simulink model "MPC_planner_201105"  (R2020a)
settings: Solver=VariableStepAuto  StartTime=0  StopTime=30  FixedStep=0.001  RelTol=1e-3  AbsTol=1e-6
InitFcn:
  | Lw = 1.6;
  | lf = 1.4;
  | lr = 1.65;
values from neighbouring files (symbols this model uses):
  pos_error_max = 0.1    [nmpc_design.m]
  v_error_max = 0.12    [nmpc_design.m]
  yaw_error_max = 1.8*pi/180    (= 0.0314159265359)    [nmpc_design.m]
libraries: Solver_SF x1, mpclib x1
settings Model: ExtModeTrigMode=oneshot  ExtModeArmWhenConnect=off  OrderedModelArguments=off  Creator=ywata  LastModifiedBy=cksgh
settings SolverCC: AutoScaleAbsTol=off  AlgebraicLoopSolver=LineSearch
settings DataIOCC: SaveFormat=Array  ReturnWorkspaceOutputs=off  SignalLoggingName=sigsOut
settings OptimizationCC: BlockReduction=off  BooleanDataType=off  LifeSpan=inf
settings DebuggingCC: SaveWithParameterizedLinksMsg=none  UnderspecifiedInitializationDetection=Classic  MergeDetectMultiDrivingBlocksExec=none  SignalResolutionControl=TryResolveAllWithWarning  MultiTaskDSMMsg=warning  MultiTaskCondExecSysMsg=none  FcnCallInpInsideContextMsg=warning  StateNameClashWarn=warning  SFUnexpectedBacktrackingDiag=warning  SFNoUnconditionalDefaultTransitionDiag=warning  UnderSpecifiedDimensionMsg=warning  ArithmeticOperatorsInVariantConditions=warning
settings HardwareCC: ProdBitPerPointer=32  ProdBitPerSizeT=32  ProdBitPerPtrDiffT=32  ProdLargestAtomicFloat=None  ProdIntDivRoundTo=Undefined  ProdEndianess=Unspecified  ProdWordSize=32  ProdHWDeviceType=32-bit Generic  TargetUnknown=on
settings ModelReferenceCC: PropagateSignalLabelsOutOfModel=off
settings SFSimCC: SimUseLocalCustomCode=off  CustomCodeUndefinedFunction=UseInterfaceOnly
settings RTWCC: TemplateMakefile=grt_vc.tmf  RTWUseLocalCustomCode=off
settings CodeAppCC: StateflowObjectComments=on
settings GRTTargetCC: TargetFcnLib=ansi_tfl_tmw.mat  TargetLangStandard=C89/C90 (ANSI)  CombineOutputUpdateFcns=off  GRTInterface=on
settings ConfigComp: CovMetricSettings=dw  CovHtmlReporting=on  CovSaveCumulativeToWorkspaceVar=on  CovSaveSingleToWorkspaceVar=on  CovExternalEMLEnable=off

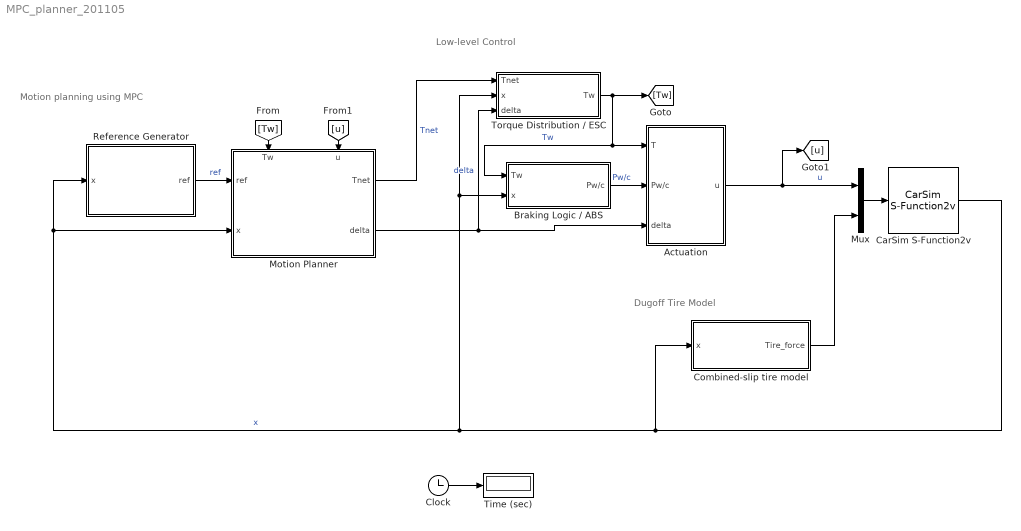
== system MPC_planner_201105 ==
  note: Dugoff Tire Model
  note: Low-level Control
  note: Motion planning using MPC
  Actuation : Subsystem
      mask Display: image('actuation_illust.png'); % Use "Edit Image" on toolstrip to change.
  Braking Logic / ABS : Subsystem
  CarSim S-Function2v : Solver_SF/CarSim S-Function2v  Priority=1  VehicleCode=i_i  SIMFILE=simfile.sim
      settings: AttributesFormatString=Vehicle Code: %<VehicleCode>
  Clock : Clock
  Combined-slip tire model : MATLAB Function  TreatAsAtomicUnit=on
  Motion Planner : Subsystem
      settings: PortSchema="{\"entries\":[{\"content\":{\"sides\":[{\"content\":{\"connectorIds\":[\"In1\",\"In2\"]},\"type\":\"ConnectorPlacement.EquallySpacedRectSide\",\"uuid\":\"a787b7cf-3cc5-479b-b22e-301a5134f3f2\"},{\"content\":{\"connectorIds\":[\"Out1\",\"Out2\"],\"side\":\"RIGHT\"},\"type\":\"ConnectorPlacement.EquallySpacedRectSide\",\"uuid\":\"a5bbac53-00df-45df-8e98-5eeb23656513\"},{\"content\":{\"connectorIds\":[\"In3\",\"In4\"],\"side\":\"TOP\"},\"type\":\"ConnectorPlacement.EquallySpacedRectSide\",\"uuid\":\"33a2ca21-4178-496c-88bb-777b57c1de4f\"}]},\"type\":\"ConnectorPlacement.EquallySpacedConnector\",\"uuid\":\"b7e07e24-f75d-4d53-b2e7-cf41caae1095\"}],\"packageUris\":[\"http://schema.mathworks.com/mf0/Connector/19700101\"],\"version\":\"1.0\"}"
      mask Display: image('mpc_illust.png'); % Use "Edit Image" on toolstrip to change.
  Mux : Mux  Inputs=[10 8]
  Reference Generator : Subsystem
      mask Display: image('refGen_illust.png'); % Use "Edit Image" on toolstrip to change.
  Time (sec) : Display
      settings: Format=bank  Decimation=100
  Torque Distribution / ESC : Subsystem
  wires:
  Clock/1 -> Time (sec)/1
  CarSim S-Function2v/1 -> Reference Generator/1(x), Motion Planner/2(x), Torque Distribution / ESC/2(x), Braking Logic / ABS/2(x), Combined-slip tire model/1(x)  "x"
  Reference Generator/1(ref) -> Motion Planner/1(ref)  "ref"
  Torque Distribution / ESC/1(Tw) -> [Tw], Actuation/1(T), Braking Logic / ABS/1(Tw)  "Tw"
  Braking Logic / ABS/1(Pw/c) -> Actuation/2(Pw/c)  "Pw/c"
  Mux/1 -> CarSim S-Function2v/1
  Actuation/1(u) -> [u], Mux/1  "u"
  Combined-slip tire model/1(Tire_force) -> Mux/2
  [u] -> Motion Planner/4(u)
  [Tw] -> Motion Planner/3(Tw)
  Motion Planner/2(delta) -> Torque Distribution / ESC/3(delta), Actuation/3(delta)  "delta"
  Motion Planner/1(Tnet) -> Torque Distribution / ESC/1(Tnet)  "Tnet"

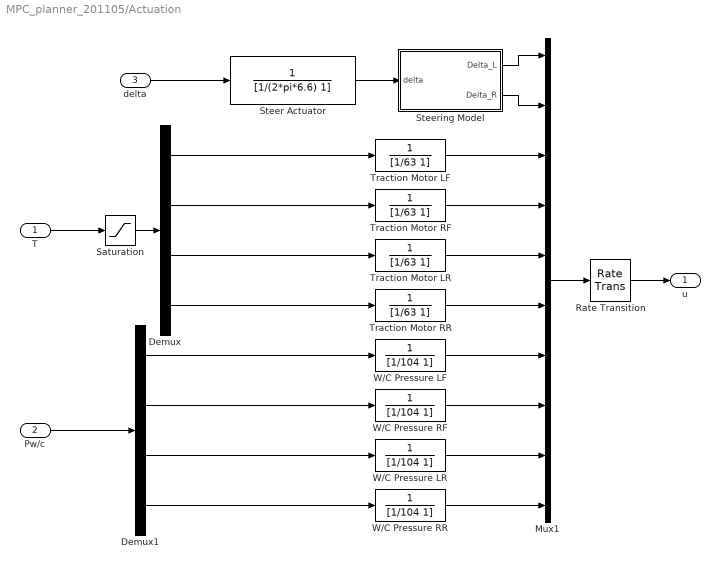
== system MPC_planner_201105/Actuation ==
  T : Inport
  Pw/c : Inport  Port=2
  delta : Inport  Port=3
  Demux : Demux
  Demux1 : Demux
  Mux1 : Mux  Inputs=10
  Rate Transition : RateTransition
  Saturation : Saturate  UpperLimit=650  LowerLimit=0
  Steer Actuator : TransferFcn  Denominator=[1/(2*pi*6.6) 1]
  Steering Model : Subsystem
  Traction Motor LF : TransferFcn  Denominator=[1/63 1]
  Traction Motor LR : TransferFcn  Denominator=[1/63 1]
  Traction Motor RF : TransferFcn  Denominator=[1/63 1]
  Traction Motor RR : TransferFcn  Denominator=[1/63 1]
  W/C Pressure LF : TransferFcn  Denominator=[1/104 1]
  W/C Pressure LR : TransferFcn  Denominator=[1/104 1]
  W/C Pressure RF : TransferFcn  Denominator=[1/104 1]
  W/C Pressure RR : TransferFcn  Denominator=[1/104 1]
  u : Outport
  wires:
  Rate Transition/1 -> u/1
  Traction Motor RR/1 -> Mux1/6
  Traction Motor LR/1 -> Mux1/5
  Traction Motor LF/1 -> Mux1/3
  Steering Model/2(Delta_R) -> Mux1/2
  Steering Model/1(Delta_L) -> Mux1/1
  Traction Motor RF/1 -> Mux1/4
  delta/1 -> Steer Actuator/1
  Mux1/1 -> Rate Transition/1
  Demux/1 -> Traction Motor LF/1
  Demux/2 -> Traction Motor RF/1
  Demux/3 -> Traction Motor LR/1
  Demux/4 -> Traction Motor RR/1
  Demux1/2 -> W/C Pressure RF/1
  W/C Pressure LF/1 -> Mux1/7
  W/C Pressure RF/1 -> Mux1/8
  W/C Pressure LR/1 -> Mux1/9
  W/C Pressure RR/1 -> Mux1/10
  Demux1/3 -> W/C Pressure LR/1
  Demux1/1 -> W/C Pressure LF/1
  Demux1/4 -> W/C Pressure RR/1
  Pw/c/1 -> Demux1/1
  Saturation/1 -> Demux/1
  T/1 -> Saturation/1
  Steer Actuator/1 -> Steering Model/1(delta)

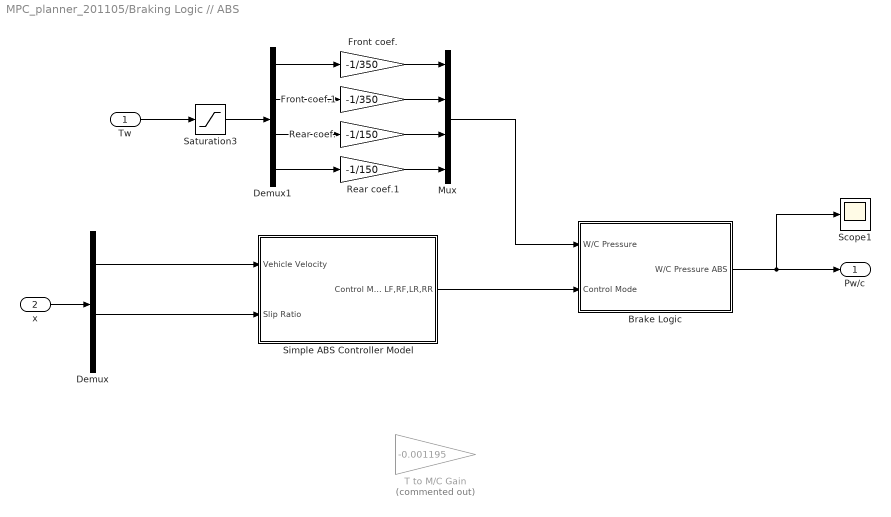
== system MPC_planner_201105/Braking Logic // ABS ==
  Tw : Inport
  x : Inport  Port=2
  "Brake Logic " : Subsystem
  Demux : Demux  Outputs=[5 1 3 4 1 4]
  Demux1 : Demux
  Front coef. : Gain  Gain=-1/350
  Front coef.1 : Gain  Gain=-1/350
  Mux : Mux
  Rear coef. : Gain  Gain=-1/150
  Rear coef.1 : Gain  Gain=-1/150
  Saturation3 : Saturate  UpperLimit=0  LowerLimit=-2300/4
  Scope1 : Scope
  Simple ABS Controller Model : Subsystem
  T to M/C Gain : Gain  Commented=on  Gain=-0.001195
  Pw/c : Outport
  wires:
  x/1 -> Demux/1
  Mux/1 -> "Brake Logic "/1(W/C Pressure)
  Demux/2 -> Simple ABS Controller Model/1(Vehicle Velocity)
  Demux/4 -> Simple ABS Controller Model/2(Slip Ratio)
  Simple ABS Controller Model/1(Control Mode LF,RF,LR,RR) -> "Brake Logic "/2(Control Mode)
  Tw/1 -> Saturation3/1
  Front coef.1/1 -> Mux/2
  Front coef./1 -> Mux/1
  Rear coef./1 -> Mux/3
  Rear coef.1/1 -> Mux/4
  Demux1/1 -> Front coef./1
  Demux1/2 -> Front coef.1/1
  Demux1/3 -> Rear coef./1
  Demux1/4 -> Rear coef.1/1
  "Brake Logic "/1(W/C Pressure ABS) -> Scope1/1, Pw/c/1
  Saturation3/1 -> Demux1/1

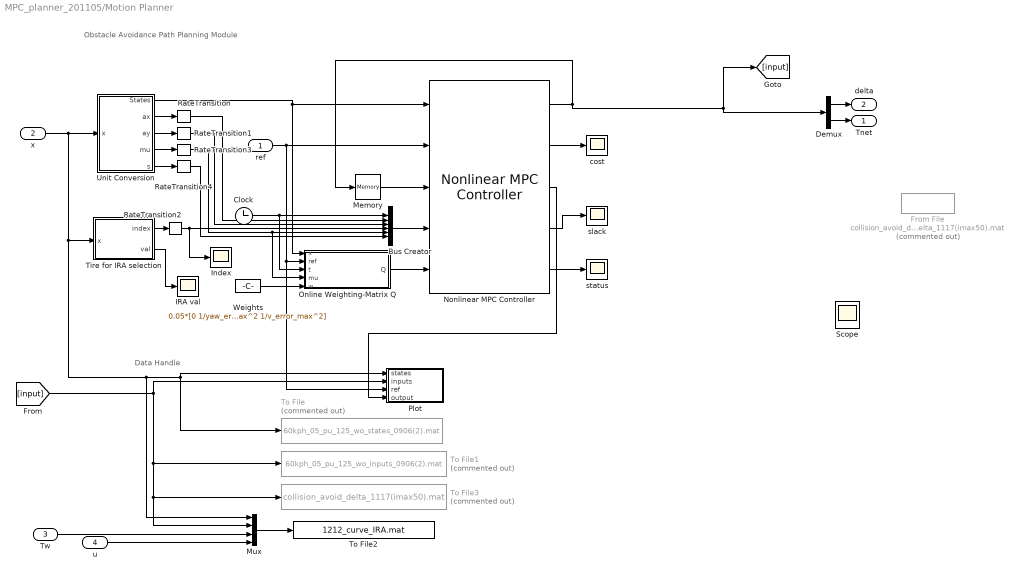
== system MPC_planner_201105/Motion Planner ==
  note: Data Handle
  note: Obstacle Avoidance Path Planning Module
  ref : Inport
  x : Inport  Port=2
  Tw : Inport  Port=3
  u : Inport  Port=4
  Bus Creator : BusCreator  Inputs=6  OutDataTypeStr=Bus: myBusObject  NonVirtualBus=on
      settings: InheritFromInputs=off
  Clock : Clock
  Demux : Demux  Outputs=2
  From File : FromFile  Commented=on  FileName=collision_avoid_delta_1117(imax50).mat  SampleTime=0
  IRA val : Scope
  Index : Scope
  Memory : Memory  InitialCondition=[0 100]  InheritSampleTime=on
  Mux : Mux
  Nonlinear MPC Controller : mpclib/Nonlinear MPC Controller  SCDEnableBlockLinearizationSpecification=on  nlmpcobj=nlobj  UseObjectTs=on  UseMEX=off  md_enabled=off  mvtarget_enabled=off  param_enabled=on  cost_enabled=on  mvseq_enabled=off  stateseq_enabled=off  ovseq_enabled=on  slack_enabled=on  status_enabled=on  ov_min=off  ov_max=off  mv_min=off  mv_max=off  mvrate_min=off  mvrate_max=off  state_min=off  state_max=off  ov_weight=on  mv_weight=off  mvrate_weight=off  ecr_weight=off  nlp_initialize=off
  Online Weighting-Matrix Q : MATLAB Function  TreatAsAtomicUnit=on  SystemSampleTime=0.05
  Plot : Subsystem
  RateTransition : RateTransition
  RateTransition1 : RateTransition
  RateTransition2 : RateTransition  InitialCondition=1
  RateTransition3 : RateTransition  InitialCondition=0.9
  RateTransition4 : RateTransition  InitialCondition=[0 0 0 0]'
  Scope : Scope
  Tire for IRA selection : MATLAB Function  TreatAsAtomicUnit=on
  To File : ToFile  Commented=on  Filename=60kph_05_pu_125_wo_states_0906(2).mat  MatrixName=states  SaveFormat=Timeseries
  To File1 : ToFile  Commented=on  Filename=60kph_05_pu_125_wo_inputs_0906(2).mat  MatrixName=inputs  SaveFormat=Timeseries
  To File2 : ToFile  Filename=1212_curve_IRA.mat  MatrixName=data  SaveFormat=Timeseries
  To File3 : ToFile  Commented=on  Filename=collision_avoid_delta_1117(imax50).mat  MatrixName=inputs  SaveFormat=Timeseries
  Unit Conversion : Subsystem
  Weights : Constant  Value=0.05*[0 1/yaw_error_max^2 1/pos_error_max^2 1/pos_error_max^2 1/v_error_max^2]
  cost : Scope
  slack : Scope
  status : Scope
  Tnet : Outport
  delta : Outport  Port=2
  wires:
  Memory/1 -> Nonlinear MPC Controller/3
  ref/1 -> Plot/3(ref), Online Weighting-Matrix Q/2(ref), Nonlinear MPC Controller/2
  Unit Conversion/1(States) -> Online Weighting-Matrix Q/1(x), Nonlinear MPC Controller/1
  Nonlinear MPC Controller/5 -> status/1
  Nonlinear MPC Controller/2 -> cost/1
  Clock/1 -> Online Weighting-Matrix Q/3(t), Bus Creator/1
  RateTransition/1 -> Bus Creator/2
  RateTransition1/1 -> Bus Creator/3
  Unit Conversion/4(mu) -> RateTransition3/1
  Bus Creator/1 -> Nonlinear MPC Controller/4
  Unit Conversion/2(ax) -> RateTransition/1
  Weights/1 -> Online Weighting-Matrix Q/5(w)
  x/1 -> Mux/1, To File/1, Plot/1(states), Tire for IRA selection/1(x), Unit Conversion/1(x)
  Unit Conversion/3(ay) -> RateTransition1/1
  RateTransition2/1 -> Index/1, Bus Creator/4
  Nonlinear MPC Controller/4 -> slack/1
  Demux/2 -> Tnet/1
  Demux/1 -> delta/1
  Nonlinear MPC Controller/1 -> Demux/1, [input], Memory/1
  [input] -> Mux/2, To File3/1, To File1/1, Plot/2(inputs)
  RateTransition3/1 -> Online Weighting-Matrix Q/4(mu), Bus Creator/5
  Unit Conversion/5(s) -> RateTransition4/1
  RateTransition4/1 -> Bus Creator/6
  Mux/1 -> To File2/1
  Tire for IRA selection/1(index) -> RateTransition2/1
  Tw/1 -> Mux/3
  u/1 -> Mux/4
  Online Weighting-Matrix Q/1(Q) -> Nonlinear MPC Controller/5
  Nonlinear MPC Controller/3 -> Plot/4(output)
  Tire for IRA selection/2(val) -> IRA val/1

== system MPC_planner_201105/Reference Generator ==
  x : Inport
  MATLAB Function : MATLAB Function  TreatAsAtomicUnit=on  SystemSampleTime=0.05
  Spline curve from workspace : FromWorkspace  Commented=on  VariableName=s
  ref : Outport
  wires:
  MATLAB Function/1(ref) -> ref/1
  x/1 -> MATLAB Function/1(state)

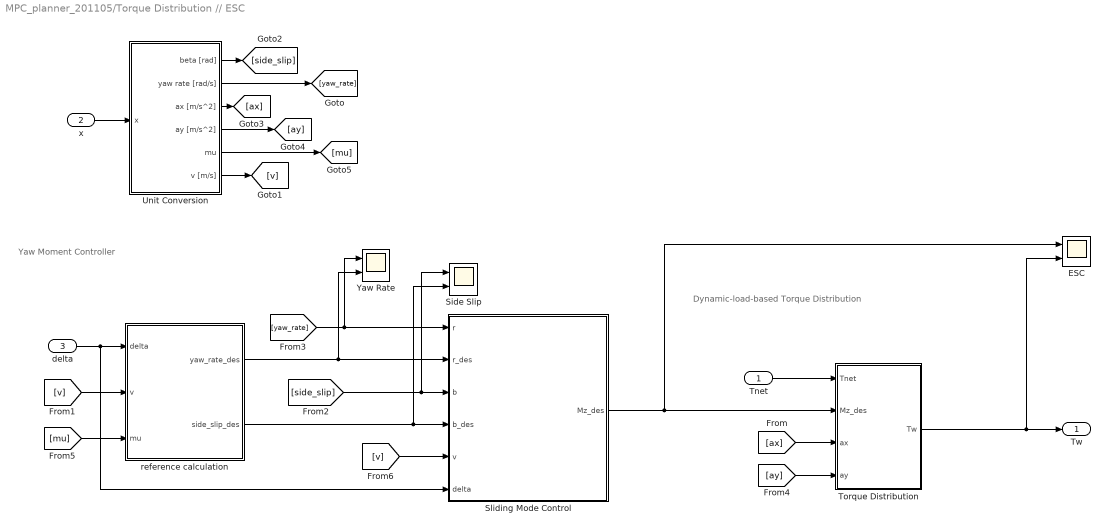
== system MPC_planner_201105/Torque Distribution // ESC ==
  note: Dynamic-load-based Torque Distribution
  note: Yaw Moment Controller
  Tnet : Inport
  x : Inport  Port=2
  delta : Inport  Port=3
  ESC : Scope  NumInputPorts=2
  Side Slip : Scope  NumInputPorts=2
  Sliding Mode Control : MATLAB Function  TreatAsAtomicUnit=on
  Torque Distribution : MATLAB Function  TreatAsAtomicUnit=on
  Unit Conversion : Subsystem
  Yaw Rate : Scope  NumInputPorts=2
  reference calculation : MATLAB Function  TreatAsAtomicUnit=on
  Tw : Outport
  wires:
  [yaw_rate] -> Yaw Rate/1, Sliding Mode Control/1(r)
  delta/1 -> reference calculation/1(delta), Sliding Mode Control/6(delta)
  reference calculation/2(side_slip_des) -> Side Slip/2, Sliding Mode Control/4(b_des)
  reference calculation/1(yaw_rate_des) -> Yaw Rate/2, Sliding Mode Control/2(r_des)
  [side_slip] -> Side Slip/1, Sliding Mode Control/3(b)
  [v] -> reference calculation/2(v)
  x/1 -> Unit Conversion/1(x)
  Unit Conversion/2(yaw rate [rad/s]) -> [yaw_rate]
  Unit Conversion/1(beta [rad]) -> [side_slip]
  Unit Conversion/3(ax [m/s^2]) -> [ax]
  Unit Conversion/4(ay [m/s^2]) -> [ay]
  [ay] -> Torque Distribution/4(ay)
  [ax] -> Torque Distribution/3(ax)
  Torque Distribution/1(Tw) -> ESC/2, Tw/1
  Tnet/1 -> Torque Distribution/1(Tnet)
  Unit Conversion/5(mu) -> [mu]
  [mu] -> reference calculation/3(mu)
  Unit Conversion/6(v [m/s]) -> [v]
  [v] -> Sliding Mode Control/5(v)
  Sliding Mode Control/1(Mz_des) -> Torque Distribution/2(Mz_des), ESC/1

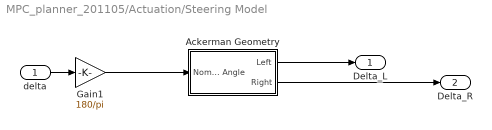
== system MPC_planner_201105/Actuation/Steering Model ==
  delta : Inport
  Ackerman Geometry : Subsystem
  Gain1 : Gain  Gain=180/pi
  Delta_L : Outport
  Delta_R : Outport  Port=2
  wires:
  Ackerman Geometry/2(Right) -> Delta_R/1
  Gain1/1 -> Ackerman Geometry/1(Nominal Angle)
  Ackerman Geometry/1(Left) -> Delta_L/1
  delta/1 -> Gain1/1

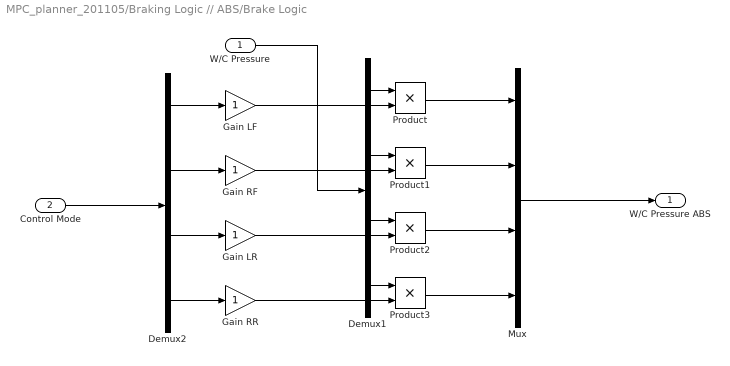
== system MPC_planner_201105/Braking Logic // ABS/Brake Logic  ==
  W/C Pressure : Inport
  Control Mode : Inport  Port=2
  Demux1 : Demux
  Demux2 : Demux
  Gain LF : Gain
  Gain LR : Gain
  Gain RF : Gain
  Gain RR : Gain
  Mux : Mux
  Product{,1..3} (4 alike) : Product
  W/C Pressure ABS : Outport
  wires:
  Demux2/1 -> Gain LF/1
  Demux2/4 -> Gain RR/1
  Demux2/3 -> Gain LR/1
  Gain LR/1 -> Product2/2
  Mux/1 -> W/C Pressure ABS/1
  Gain RF/1 -> Product1/2
  Gain RR/1 -> Product3/2
  Demux2/2 -> Gain RF/1
  Gain LF/1 -> Product/2
  Control Mode/1 -> Demux2/1
  Product/1 -> Mux/1
  Product1/1 -> Mux/2
  Product2/1 -> Mux/3
  Product3/1 -> Mux/4
  Demux1/1 -> Product/1
  Demux1/2 -> Product1/1
  Demux1/3 -> Product2/1
  Demux1/4 -> Product3/1
  W/C Pressure/1 -> Demux1/1

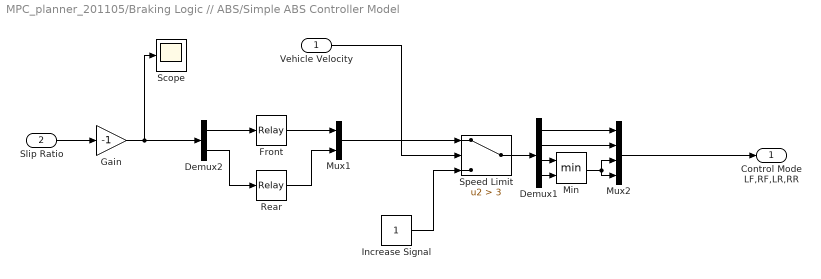
== system MPC_planner_201105/Braking Logic // ABS/Simple ABS Controller Model ==
  Vehicle Velocity : Inport
  Slip Ratio : Inport  Port=2
  Demux1 : Demux
  Demux2 : Demux  Outputs=[2 2]
  Front : Relay  OnSwitchValue=0.1  OffSwitchValue=0.05  OnOutputValue=0  OffOutputValue=1
  Gain : Gain  Gain=-1
  Increase Signal : Constant
  Min : MinMax  Inputs=2
  Mux1 : Mux  Inputs=2
  Mux2 : Mux
  Rear : Relay  OnSwitchValue=0.1  OffSwitchValue=0.05  OnOutputValue=0  OffOutputValue=1
  Scope : Scope
  Speed Limit : Switch  Criteria=u2 > Threshold  Threshold=3
  Control Mode LF,RF,LR,RR : Outport
  wires:
  Front/1 -> Mux1/1
  Speed Limit/1 -> Demux1/1
  Min/1 -> Mux2/3, Mux2/4
  Mux1/1 -> Speed Limit/1
  Increase Signal/1 -> Speed Limit/3
  Demux1/2 -> Mux2/2
  Demux1/4 -> Min/2
  Vehicle Velocity/1 -> Speed Limit/2
  Rear/1 -> Mux1/2
  Demux1/3 -> Min/1
  Demux1/1 -> Mux2/1
  Mux2/1 -> Control Mode LF,RF,LR,RR/1
  Slip Ratio/1 -> Gain/1
  Demux2/1 -> Front/1
  Demux2/2 -> Rear/1
  Gain/1 -> Scope/1, Demux2/1

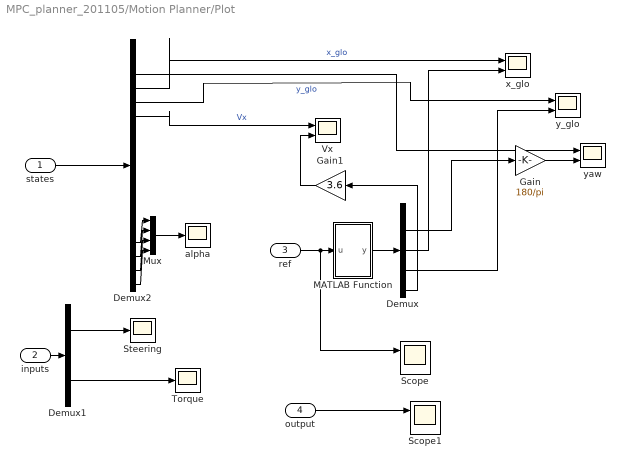
== system MPC_planner_201105/Motion Planner/Plot ==
  states : Inport
  inputs : Inport  Port=2
  ref : Inport  Port=3
  output : Inport  Port=4
  Demux : Demux  Outputs=5
  Demux1 : Demux  Outputs=2
  Demux2 : Demux  Outputs=18
  Gain : Gain  Gain=180/pi
  Gain1 : Gain  Gain=3.6
  MATLAB Function : MATLAB Function  TreatAsAtomicUnit=on
  Mux : Mux
  Scope : Scope  NumInputPorts=2
  Scope1 : Scope  NumInputPorts=2
  Steering : Scope
  Torque : Scope
  Vx : Scope  NumInputPorts=2
  alpha : Scope
  x_glo : Scope  NumInputPorts=2
  y_glo : Scope  NumInputPorts=2
  yaw : Scope  NumInputPorts=2
  wires:
  states/1 -> Demux2/1
  Demux2/5 -> y_glo/1  "y_glo"
  Demux2/6 -> Vx/1  "Vx"
  inputs/1 -> Demux1/1
  Demux1/1 -> Steering/1
  Demux1/2 -> Torque/1
  Demux2/15 -> Mux/1
  Demux2/16 -> Mux/2
  Demux2/17 -> Mux/3
  Demux2/18 -> Mux/4
  Mux/1 -> alpha/1
  Demux/4 -> y_glo/2
  MATLAB Function/1(y) -> Demux/1
  ref/1 -> Scope/1, MATLAB Function/1(u)
  Demux2/3 -> yaw/1
  Demux/2 -> Gain/1
  Demux2/4 -> x_glo/1  "x_glo"
  Demux/3 -> x_glo/2
  Gain/1 -> yaw/2
  Demux/5 -> Gain1/1
  Gain1/1 -> Vx/2
  output/1 -> Scope1/1

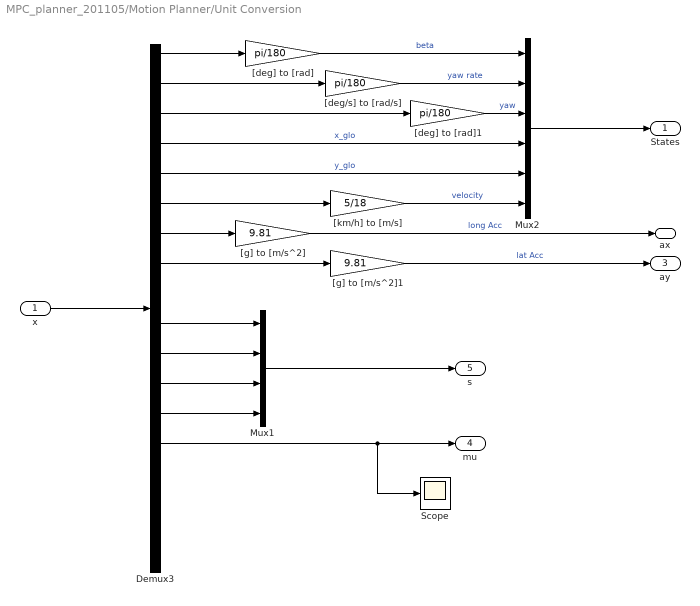
== system MPC_planner_201105/Motion Planner/Unit Conversion ==
  x : Inport
  Demux3 : Demux  Outputs=18
  Mux1 : Mux
  Mux2 : Mux  Inputs=6
  Scope : Scope
  "[deg/s] to [rad/s]" : Gain  Gain=pi/180
  "[deg] to [rad]" : Gain  Gain=pi/180
  "[deg] to [rad]1" : Gain  Gain=pi/180
  "[g] to [m/s^2]" : Gain  Gain=9.81
  "[g] to [m/s^2]1" : Gain  Gain=9.81
  "[km/h] to [m/s]" : Gain  Gain=5/18
  States : Outport
  ax : Outport  Port=2
  ay : Outport  Port=3
  mu : Outport  Port=4
  s : Outport  Port=5
  wires:
  Demux3/1 -> "[deg] to [rad]"/1
  x/1 -> Demux3/1
  "[km/h] to [m/s]"/1 -> Mux2/6  "velocity"
  Mux2/1 -> States/1
  Demux3/6 -> "[km/h] to [m/s]"/1
  "[deg] to [rad]"/1 -> Mux2/1  "beta"
  Demux3/2 -> "[deg/s] to [rad/s]"/1
  "[deg/s] to [rad/s]"/1 -> Mux2/2  "yaw rate"
  Demux3/3 -> "[deg] to [rad]1"/1
  "[deg] to [rad]1"/1 -> Mux2/3  "yaw"
  Demux3/4 -> Mux2/4  "x_glo"
  Demux3/5 -> Mux2/5  "y_glo"
  Demux3/7 -> "[g] to [m/s^2]"/1
  "[g] to [m/s^2]"/1 -> ax/1  "long Acc"
  Demux3/8 -> "[g] to [m/s^2]1"/1
  "[g] to [m/s^2]1"/1 -> ay/1  "lat Acc"
  Demux3/14 -> Scope/1, mu/1
  Demux3/10 -> Mux1/1
  Demux3/11 -> Mux1/2
  Demux3/12 -> Mux1/3
  Demux3/13 -> Mux1/4
  Mux1/1 -> s/1

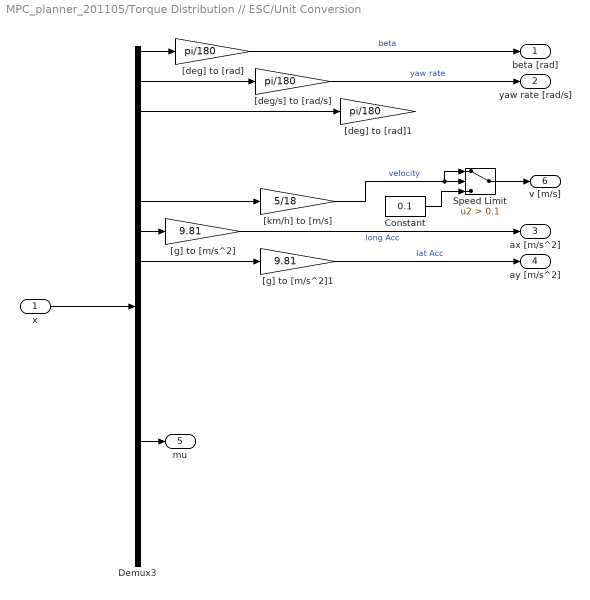
== system MPC_planner_201105/Torque Distribution // ESC/Unit Conversion ==
  x : Inport
  Constant : Constant  Value=0.1
  Demux3 : Demux  Outputs=18
  Speed Limit : Switch  Criteria=u2 > Threshold  Threshold=0.1
  "[deg/s] to [rad/s]" : Gain  Gain=pi/180
  "[deg] to [rad]" : Gain  Gain=pi/180
  "[deg] to [rad]1" : Gain  Gain=pi/180
  "[g] to [m/s^2]" : Gain  Gain=9.81
  "[g] to [m/s^2]1" : Gain  Gain=9.81
  "[km/h] to [m/s]" : Gain  Gain=5/18
  beta [rad] : Outport
  yaw rate [rad/s] : Outport  Port=2
  ax [m/s^2] : Outport  Port=3
  ay [m/s^2] : Outport  Port=4
  mu : Outport  Port=5
  v [m/s] : Outport  Port=6
  wires:
  Demux3/1 -> "[deg] to [rad]"/1
  x/1 -> Demux3/1
  "[km/h] to [m/s]"/1 -> Speed Limit/1, Speed Limit/2  "velocity"
  Demux3/6 -> "[km/h] to [m/s]"/1
  "[deg] to [rad]"/1 -> beta [rad]/1  "beta"
  Demux3/2 -> "[deg/s] to [rad/s]"/1
  "[deg/s] to [rad/s]"/1 -> yaw rate [rad/s]/1  "yaw rate"
  Demux3/3 -> "[deg] to [rad]1"/1
  Demux3/7 -> "[g] to [m/s^2]"/1
  "[g] to [m/s^2]"/1 -> ax [m/s^2]/1  "long Acc"
  Demux3/8 -> "[g] to [m/s^2]1"/1
  "[g] to [m/s^2]1"/1 -> ay [m/s^2]/1  "lat Acc"
  Demux3/14 -> mu/1
  Constant/1 -> Speed Limit/3
  Speed Limit/1 -> v [m/s]/1

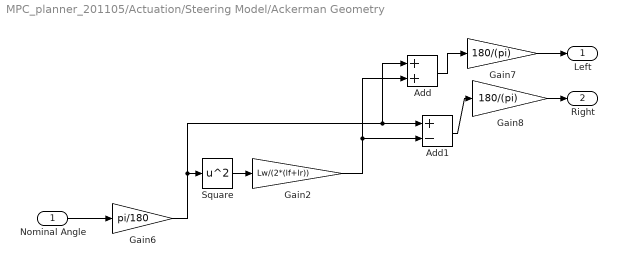
== system MPC_planner_201105/Actuation/Steering Model/Ackerman Geometry ==
  Nominal Angle : Inport
  Add : Sum
  Add1 : Sum  Inputs=+-
  Gain2 : Gain  Gain=Lw/(2*(lf+lr))
  Gain6 : Gain  Gain=pi/180
  Gain7 : Gain  Gain=180/(pi)
  Gain8 : Gain  Gain=180/(pi)
  Square : Math  Operator=square  SignedPower=on  SaturateOnIntegerOverflow=on
  Left : Outport
  Right : Outport  Port=2
  wires:
  Square/1 -> Gain2/1
  Gain6/1 -> Add/1, Add1/1, Square/1
  Add/1 -> Gain7/1
  Add1/1 -> Gain8/1
  Nominal Angle/1 -> Gain6/1
  Gain7/1 -> Left/1
  Gain8/1 -> Right/1
  Gain2/1 -> Add1/2, Add/2

== matlab function MPC_planner_201105/Torque Distribution // ESC/Sliding Mode Control ==
  data: r input; Mz_des output; r_des input; b input; b_des input; v input; delta input
function Mz_des  = fcn(r,r_des,b,b_des, v, delta)

m = 1650 + 180; % Sprung mass and unsprung mass
Iz = 3234;
lf = 1.4;
lr = 1.65;

% norminal cornering stiffness [N/rad]
Cf = -(1305.3)*180/pi/7; % Fzf = 4856*2 N
Cr = -(1122.7)*180/pi/7; % Fzr = 4140*2 N


% Yaw moment input based on sliding mode control
rho = 0.001;
K = 3;
theta = 100;
a11 = -2*(Cf+Cr)/(m*v);
a12 = -1-2*(lf*Cf-lr*Cr)/(m*v^2);
a21 = -2*(lf*Cf-lr*Cr)/Iz;
a22 = -2*(lf^2*Cf+lr^2*Cr)/(Iz*v);

Mz_eq = -Iz*(rho*a11+a21)*b-Iz*(rho*a12+a22)*r-Iz*(rho*2*Cf/m/v+2*lf*Cf/Iz)*delta;
% Mz_eq = -Iz*(a21*b+a22*r+2*lf*Cf/Iz)*delta;
e = ((r-r_des) +rho*(b-b_des) ) / theta;
if abs(e) > 1
    e = sign(e);
end

Mz_des = Mz_eq - Iz*(K*e);
% Mz_des = Mz_des*0.001;

== matlab function MPC_planner_201105/Torque Distribution // ESC/reference calculation ==
  data: delta input; yaw_rate_des output; v input; side_slip_des output; mu input
function [yaw_rate_des, side_slip_des] = fcn(delta, v, mu)

m = 1650 + 180; % Sprung mass and unsprung mass
g = 9.81;
lf = 1.4;
lr = 1.65;
L = lf+lr;

% cornering stiffness [N/rad]
Cf = -1305.3 * 180/pi/7; % Fzf = 4856*2 N
Cr = -1122.7 * 180/pi/7; % Fzr = 4140*2 N

% desired Yaw rate and Side slip
yaw_rate_des = sign(delta)*abs(v/(lf+lr+ (m*v^2*(lr*Cr-lf*Cf)/(2*Cf*Cr*L)) )*delta); % [rad/s]
side_slip_des = sign(delta)*abs((lr-lf*m*v^2/(2*Cr*L))/(L+(m*v^2*(lr*Cr-lf*Cf)/(2*Cf*Cr*L)))*delta); % [rad]

% upper bounnd
yaw_rate_ub = abs(0.85*mu*g/v);
side_slip_ub = abs(atan(0.02*mu*9.81));

if abs(yaw_rate_des) > yaw_rate_ub
    yaw_rate_des = sign(delta)*yaw_rate_ub;
end
if abs(side_slip_des) > side_slip_ub
    side_slip_des = sign(delta)*side_slip_ub;
end
side_slip_des = -side_slip_des;

== matlab function MPC_planner_201105/Motion Planner/Online Weighting-Matrix Q ==
  data: x input; ref input; t input; mu input; Q output; w input
function Q = fcn(x,ref,t,mu,w)
x_ref = ref(:,3);
y_ref = ref(:,4);
V = x(6);
g = 9.81;
p = 20;
Ts = 0.05;

af = 6*sqrt(2)/2; b = 3*sqrt(2)/2;
d = V.^2/mu/g - 2;
v_obs = 50/3.6;
x_ini = 70;
x_obs_cur = x_ini + t*v_obs;

%%%% Moving obstacle %%%%
% x_obs = (x_obs_cur+v_obs*Ts: v_obs*Ts :x_obs_cur + v_obs*Ts*p)';
% if x_ref(1) < x_obs_cur
%     K_mv = ( (x_ref - x_obs).^2./d.^2 + (y_ref+2).^2./b^2 ).^0.5 - 1;
%     J_mv = (exp(-0.1*K_mv)./max(K_mv,1e-2));
% else
%     K_mv = ( (x_ref - x_obs).^2./af.^2 + (y_ref+2).^2./b^2 ).^0.5 - 1;
%     J_mv = (exp(-0.1*K_mv)./max(K_mv,1e-2));
% end
%%%%%%%%%%%%%%%%%%%%%%%%%%
p_obs = [70 -2];

%%%% Pop-up obstacle %%%%
J_mv = zeros(p,1);
% if x_ref(1) > 70-2-44.444
%     if x_ref(1) < x_obs_cur
%         d = 70 - x_ref(1) -2 ;
%         K_mv = ( (x_ref - p_obs(1)).^2./d.^2 + (y_ref - p_obs(2)).^2./b^2 ).^0.5 - 1;
%         J_mv = 0.1*(exp(-10*K_mv)./max(K_mv,1e-7));
%     else
%         K_mv = ( (x_ref - p_obs(1)).^2./af.^2 + (y_ref - p_obs(2)).^2./b^2 ).^0.5 - 1;
%         J_mv = 0.1*(exp(-10*K_mv)./max(K_mv,1e-7));
%     end
% end
%%%%%%%%%%%%%%%%%%%%%%%%



%%%%%%%%%%%%%%%%%%%%% Popup Obstacle curve %%%%%%%%%%%%%%%%%%%%%%
if y_ref(1) >= 32 %29.17
    if y_ref(1) < 52
        d = p_obs(2) - y_ref(1)-2;
        K_obs = ( (x_ref - p_obs(1)).^2./b^2 + (y_ref-p_obs(2)).^2./d^2 ).^0.5 - 1;
        J_mv = 0.1*(exp(-10*K_obs)./max(K_obs,1e-7));
    else
        K_obs = ( (x_ref - p_obs(1)).^2./b^2 + (y_ref-p_obs(2)).^2./af^2 ).^0.5 - 1;
        J_mv = 0.1*(exp(-10*K_obs)./max(K_obs,1e-7));
    end
end
%%%%%%%%%%%%%%%%%%%%%%%%%%%%%%%%%%%%%%%%%%%%%%%%%%%%%%%%%%%%
k = 1./(1+0.1*J_mv);
Q = [zeros(p,1) w(2)*ones(p,1).*k w(3)*ones(p,1).*k w(4)*ones(p,1).*k w(5)*ones(p,1)];

== matlab function MPC_planner_201105/Reference Generator/MATLAB Function ==
  data: ref output; state input
function ref = fcn(state)
Hp = 20; Ts = 0.05;
ref = zeros(Hp,5);

%%%%%%%%%%%%%%%%%%%%%%%%%%% CURVE Scenario %%%%%%%%%%%%%%%%%%%%%%%%%%%%%%%%

% Load reference data
y = load('curve_left_R50_y-s.mat');
x = load('curve_left_R50_x-s.mat');
v = load('v_profile_cur50_0.3_v-s.mat');
y = y.y;
x = x.x;
v = v.v;

% initialize
x_glo = state(4); y_glo = state(5);
s = sqrt(x_glo^2 + y_glo^2); ds = 0.01;
x_ref_init = x(int16(s/ds));
y_ref_init = y(int16(s/ds));
Hp = 20; Ts = 0.05;


% Search shortest point of reference
d = dis(x_glo,y_glo,x_ref_init,y_ref_init);
df = dis(x_glo,y_glo,x(int16(s/ds) + 2),y(int16(s/ds) + 2)); % Forward search
db = dis(x_glo,y_glo,x(int16(s/ds) - 2),y(int16(s/ds) - 2)); % Backward search
if df < d
    while( df < d)
        s = s + 4*ds;
        x_ref_init = x(int16(s/ds));
        y_ref_init = y(int16(s/ds));
        d = df;
        df = dis(x_glo,y_glo,x_ref_init,y_ref_init);
    end
elseif db < d
    while( db < d)
        s = s - 4*ds;
        x_ref_init = x(int16(s/ds));
        y_ref_init = y(int16(s/ds));
        d = db;
        db = dis(x_glo,y_glo,x_ref_init,y_ref_init);
    end
end

% Calculate References
yaw_init = atan2(y(int16(s/ds)+1) - y(int16(s/ds)),x(int16(s/ds)+1) - x(int16(s/ds)));
s = max(0.01,s);
dsdt = v(int16(s/ds))*(x_ref_init*cos(yaw_init) + y_ref_init*sin(yaw_init))/s * Ts;
s_ref = zeros(Hp+1,1); x_ref = zeros(Hp,1); y_ref = zeros(Hp,1); yaw_ref = zeros(Hp,1); v_ref = zeros(Hp,1);
s_ref(1) = s + dsdt;
for i=1:1:Hp
    x_ref(i) = x(int16(s_ref(i)/ds));
    y_ref(i) = y(int16(s_ref(i)/ds));
    yaw_ref(i) = atan2(y(int16(s_ref(i)/ds)+1) - y_ref(i),x(int16(s_ref(i)/ds)+1) - x_ref(i));
    v_ref(i) = v(int16(s_ref(i)/ds));
    dsdt = v_ref(i)*(x_ref(i)*cos(yaw_ref(i)) + y_ref(i)*sin(yaw_ref(i))) / s_ref(i) * Ts;
    s_ref(i+1) = s_ref(i) + dsdt;
end



%%%%%%%%%%%%%%%%%%%%%%%%%%%%%%%%%%%%%%%%%%%%%%%%%%%%%%%%%%%%%%%%%%%%%%%%%%%



%%%%%%%%%%%%%%%%%%%%%%%%%%% STRAIGHT Scenario %%%%%%%%%%%%%%%%%%%%%%%%%%%%%
% vx = state(6)/3.6;
% yaw = state(3)*pi/180;
% x_glo = state(4);
% dx = vx*cos(yaw) * Ts;
% 
% yaw_ref = zeros(Hp,1);
% x_ref = linspace(x_glo + dx, x_glo + dx*Hp, Hp)';
% y_ref = -2*ones(Hp,1);
% v_ref = 80/3.6*ones(Hp,1);

%%%%%%%%%%%%%%%%%%%%%%%%%%%%%%%%%%%%%%%%%%%%%%%%%%%%%%%%%%%%%%%%%%%%%%%%%%%


ref(:,2) = yaw_ref;
ref(:,3) = x_ref;
ref(:,4) = y_ref;
ref(:,5) = v_ref;

function d = dis(x1,y1,x2,y2)
d = sqrt((x1-x2)^2 + (y1-y2)^2);

== matlab function MPC_planner_201105/Torque Distribution // ESC/Torque Distribution ==
  data: Tnet input; Tw output; Mz_des input; ax input; ay input
function Tw = fcn(Tnet, Mz_des, ax, ay)

m = 1650 + 180; % Sprung mass and unsprung mass
g = 9.81;
Lw = 1.6; % Track width
lf = 1.4;
lr = 1.65;
h = 0.53;

Fzfl = (g*lr/2-ax*h/2-1*ay*lr*h/Lw+ax*ay*h^2/g/Lw)*m/(lr+lf);
Fzfr = (g*lr/2-ax*h/2+1*ay*lr*h/Lw-ax*ay*h^2/g/Lw)*m/(lr+lf);
Fzrl = (g*lf/2+ax*h/2-1.2*ay*lf*h/Lw-ax*ay*h^2/g/Lw)*m/(lr+lf);
Fzrr = (g*lf/2+ax*h/2+1.2*ay*lf*h/Lw+ax*ay*h^2/g/Lw)*m/(lr+lf);
Fz = Fzfl + Fzfr + Fzrl + Fzrr;

k = [Fzfl Fzfr Fzrl Fzrr]./Fz;

Tfl = k(1)*(Tnet - Mz_des);
Tfr = k(2)*(Tnet + Mz_des);
Trl = k(3)*(Tnet - Mz_des);
Trr = k(4)*(Tnet + Mz_des);

Tw = [Tfl;Tfr;Trl;Trr];

== matlab function MPC_planner_201105/Combined-slip tire model ==
  data: x input; Tire_force output
function Tire_force = fcn(x)

m = 1650 + 180; % Sprung mass and unsprung mass
g = 9.81;
Lw = 1.6; % Track width
lf = 1.4;
lr = 1.65;
h = 0.53;

s = x(10:13)';
mu = x(14);
alpha = -x(15:18)'*pi/180;
ax = x(7)*g;
ay = x(8)*g;

Fzfl = (g*lr/2-ax*h/2-1*ay*lr*h/Lw+ax*ay*h^2/g/Lw)*m/(lr+lf);
Fzfr = (g*lr/2-ax*h/2+1*ay*lr*h/Lw-ax*ay*h^2/g/Lw)*m/(lr+lf);
Fzrl = (g*lf/2+ax*h/2-1.2*ay*lf*h/Lw-ax*ay*h^2/g/Lw)*m/(lr+lf);
Fzrr = (g*lf/2+ax*h/2+1.2*ay*lf*h/Lw+ax*ay*h^2/g/Lw)*m/(lr+lf);
Fz = [Fzfl Fzfr Fzrl Fzrr];

[Fx, Fy, lammda] = DugoffModel(Fz, alpha, s, mu);

Tire_force = [Fx Fy];

== matlab function MPC_planner_201105/Motion Planner/Tire for IRA selection ==
  data: x input; index output; val output
function [index,val] = fcn(x)


m = 1650 + 180; % Sprung mass and unsprung mass
g = 9.81;
Lw = 1.6; % Track width
lf = 1.4;
lr = 1.65;
h = 0.53;

s = x(10:13)';
mu = x(14);
alpha = -x(15:18)'*pi/180;
ax = x(7)*g;
ay = x(8)*g;

Fzfl = (g*lr/2-ax*h/2-1*ay*lr*h/Lw+ax*ay*h^2/g/Lw)*m/(lr+lf);
Fzfr = (g*lr/2-ax*h/2+1*ay*lr*h/Lw-ax*ay*h^2/g/Lw)*m/(lr+lf);
Fzrl = (g*lf/2+ax*h/2-1.2*ay*lf*h/Lw-ax*ay*h^2/g/Lw)*m/(lr+lf);
Fzrr = (g*lf/2+ax*h/2+1.2*ay*lf*h/Lw+ax*ay*h^2/g/Lw)*m/(lr+lf);
Fz = [Fzfl Fzfr Fzrl Fzrr];

[Fx, Fy, lammda] = DugoffModel(Fz, alpha, s, mu);

val = zeros(5,1);
val(1:4) = (Fx./Fz/(mu)).^2 + (Fy./Fz/(mu*0.9)).^2;
val(5) = (ax/(mu*g))^2+(ay/(mu*0.9*g))^2;
% val(5) = 0;
[val_max, index] = max(val);

== matlab function MPC_planner_201105/Motion Planner/Plot/MATLAB Function ==
  data: u input; y output
function y = fcn(u)

y = u(1,:)';
